simulink model "test_prod_riga_riga"  (R2021b)
settings: Solver=VariableStepAuto  StartTime=0.0  StopTime=10.0  RelTol=1e-3
settings Model: Creator=adity  LastModifiedBy=adity

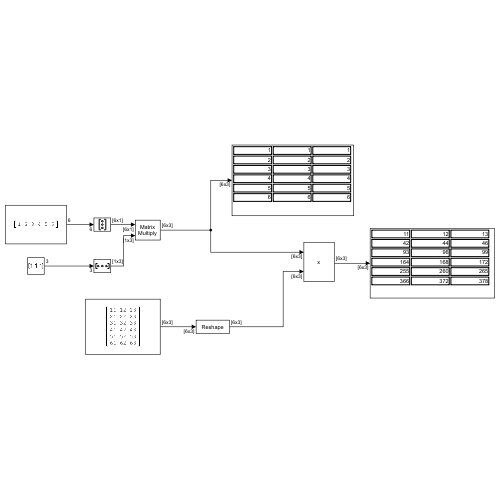
[thumbnail: Simulink's stored preview of the top-level diagram]
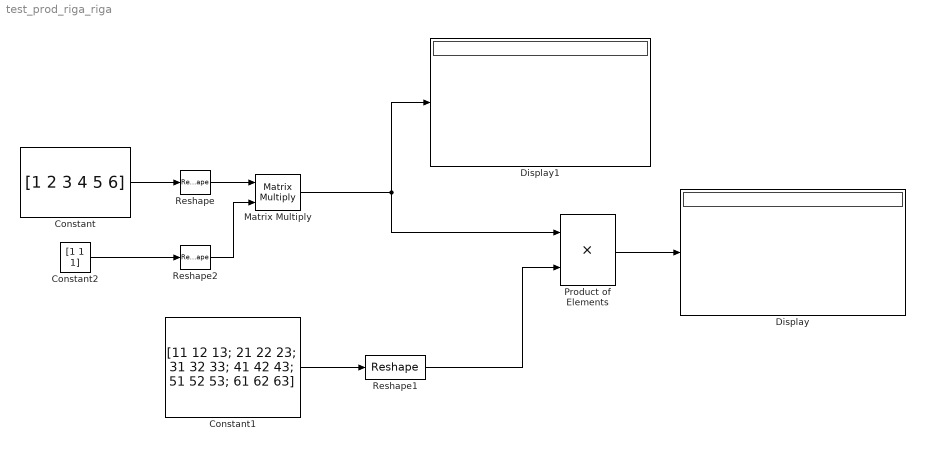
== system test_prod_riga_riga ==
  Constant : Constant  Value=[1 2 3 4 5 6]
  Constant1 : Constant  Value=[11 12 13; 21 22 23; 31 32 33; 41 42 43; 51 52 53; 61 62 63]
  Constant2 : Constant  Value=[1 1 1]
  Display : Display
  Display1 : Display
  Matrix Multiply : Product  Multiplication=Matrix(*)
  Product of Elements : Product
  Reshape : Reshape  OutputDimensionality=Column vector (2-D)
  Reshape1 : Reshape  OutputDimensionality=Customize  OutputDimensions=[6,3]
  Reshape2 : Reshape  OutputDimensionality=Row vector (2-D)
  wires:
  Constant1/1 -> Reshape1/1
  Constant/1 -> Reshape/1
  Product of Elements/1 -> Display/1
  Reshape/1 -> Matrix Multiply/1
  Constant2/1 -> Reshape2/1
  Reshape2/1 -> Matrix Multiply/2
  Matrix Multiply/1 -> Product of Elements/1, Display1/1
  Reshape1/1 -> Product of Elements/2
